simulink library "halout"  (R2021b)
settings: Solver=VariableStepAuto  StartTime=0.0  StopTime=10.0  RelTol=1e-3
undefined symbols (not defined in the file): C_TASK_5MS_S, FALSE, KHAL_CAN1TxReq_flg, KHAL_CAN2TxReq_flg, KHAL_CAN3FD3VCU1toNIDECTxReq_flg, KHAL_CAN3FD3VCU1TxReq_flg, KHAL_CAN3FD3VCU2E2E_flg, KHAL_CAN3FD3VCU2toNIDECE2E_flg, KHAL_CAN3FD3VCU2toNIDECTxReq_flg, KHAL_CAN3FD3VCU2TxReq_flg, KHAL_CAN3TxReq_flg, KHAL_CAN4FD4CE1000E2E_flg, KHAL_CAN4FD4CE1000TxReq_flg, KHAL_CAN4TxReq_flg, KHAL_CAN5TxReq_flg, KHAL_CAN7TxReq_flg, ONE_INT, TRUE, ZERO_INT
libraries: FVT_lib x258, simulink x115
(part 1 of 17)
settings Model: Creator=13168  LastModifiedBy=FVT22063
settings SolverCC: AlgebraicLoopSolver=TrustRegion
settings DataIOCC: SaveFormat=Array  SignalLoggingSaveFormat=ModelDataLogs  ReturnWorkspaceOutputs=off
settings OptimizationCC: BlockReduction=off  BooleanDataType=off
settings DebuggingCC: SaveWithParameterizedLinksMsg=none  UnderspecifiedInitializationDetection=Classic  MergeDetectMultiDrivingBlocksExec=none  SignalResolutionControl=TryResolveAllWithWarning  SFMachineParentedDataDiag=warning
settings HardwareCC: TargetUnknown=on
settings ModelReferenceCC: PropagateSignalLabelsOutOfModel=off
settings ConfigComp: CovMetricSettings=dw  CovSaveCumulativeToWorkspaceVar=on  CovSaveSingleToWorkspaceVar=on

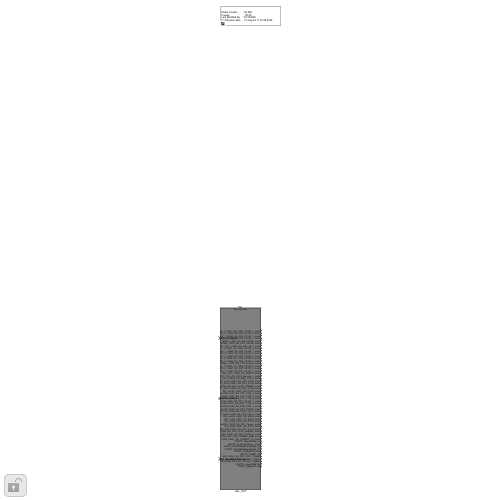
[thumbnail: Simulink's stored preview of the top-level diagram]
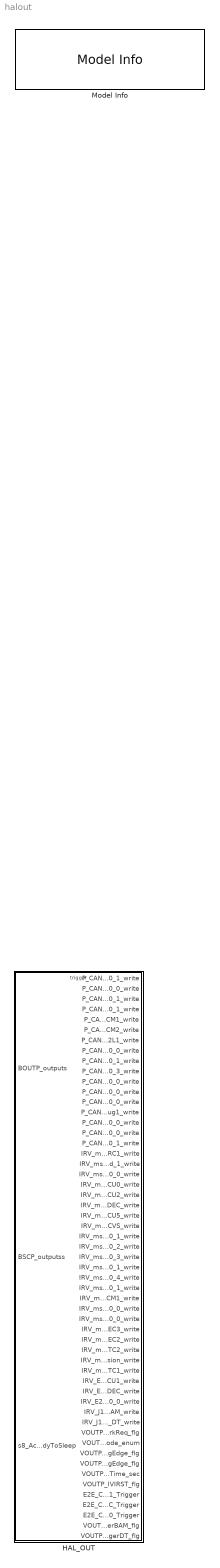
== system halout ==
  HAL_OUT : Subsystem
      settings: RTWSystemCode=Nonreusable function  RTWFcnNameOpts=Use subsystem name  RTWFileNameOpts=Use subsystem name
  Model Info : simulink/Model-Wide Utilities/Model Info  Frame=on  DisplayStringWithTags=|  HorizontalTextAlignment=Left  LeftAlignmentValue=0.02
      | Model Version        : %<ModelVersion>
      | Creator                   : %<Creator>
      | Last Modified By    : %<LastModifiedBy>
      | Modification date    : %<LastModificationDate>

== system halout/HAL_OUT ==
  BOUTP_outputs : Inport  OutDataTypeStr=Bus: BOUTP_outputs
  BSCP_outputss : Inport  Port=2  OutDataTypeStr=Bus:BSCP_outputs
  s8_AcoreReadyToSleep : Inport  Port=3
  trig_hal_out : TriggerPort  TriggerType=function-call  VariantControl=(inherit)
  Bus Selector : BusSelector  OutputSignals=VOUTP_AllCANTxReq_flg
  Bus_Selector : BusSelector  OutputSignals=VOUTP_NetworkReq_flg,VOUTP_SysPowerMode_enum,VOUTP_NvWriteReqRisingEdge_flg,VOUTP_FdcSlpReqRisingEdge_flg,VOUTP_FdcSlpTime_sec,VOUTP_triggerBAM_flg,VOUTP_triggerDT_flg
  CAN1 : Subsystem  TreatAsAtomicUnit=on
  CAN2 : Subsystem  TreatAsAtomicUnit=on
  CAN3 : Subsystem  TreatAsAtomicUnit=on
  CAN4 : Subsystem  TreatAsAtomicUnit=on
  CAN5 : Subsystem  TreatAsAtomicUnit=on
  CAN7 : Subsystem  TreatAsAtomicUnit=on
  CAN_Scheduler : Stateflow chart  TreatAsAtomicUnit=on
  Constant : Constant  Value=KHAL_CAN1TxReq_flg
  Constant1 : Constant  Value=KHAL_CAN2TxReq_flg
  Constant2 : Constant  Value=KHAL_CAN3TxReq_flg
  Constant3 : Constant  Value=KHAL_CAN4TxReq_flg
  Constant4 : Constant  Value=KHAL_CAN5TxReq_flg
  Constant5 : Constant  Value=KHAL_CAN7TxReq_flg
  Ground : Ground
  P_CAN1_GW1_C1000_1_CAN1_SG_GW1_C1000_1_write : Outport  OutDataTypeStr=Bus: DT_CAN1_SG_GW1_C1000_1
  P_CAN2_FD2_CE100_0_CAN2_SG_FD2_CE100_0_write : Outport  Port=2  OutDataTypeStr=Bus: DT_CAN2_SG_FD2_CE100_0
  P_CAN2_FD2_CE100_1_CAN2_SG_FD2_CE100_1_write : Outport  Port=3  OutDataTypeStr=Bus: DT_CAN2_SG_FD2_CE100_1
  P_CAN2_FD2_CE200_1_CAN2_SG_FD2_CE200_1_write : Outport  Port=4  OutDataTypeStr=Bus: DT_CAN2_SG_FD2_CE200_1
  P_CAN3_FD3_BCM1_CAN3_SG_FD3_BCM1_write : Outport  Port=5  OutDataTypeStr=Bus: DT_CAN3_SG_FD3_BCM1
  P_CAN3_FD3_THCM2_CAN3_SG_FD3_THCM2_write : Outport  Port=6  OutDataTypeStr=Bus: DT_CAN3_SG_FD3_THCM2
  P_CAN3_FD3_V2L1_CAN3_SG_FD3_V2L1_write : Outport  Port=7  OutDataTypeStr=Bus: DT_CAN3_SG_FD3_V2L1
  P_CAN3_GW3_CE100_0_CAN3_SG_GW3_CE100_0_write : Outport  Port=8  OutDataTypeStr=Bus: DT_CAN3_SG_GW3_CE100_0
  P_CAN4_FD4_CE100_1_CAN4_SG_FD4_CE100_1_write : Outport  Port=9  OutDataTypeStr=Bus: DT_CAN4_SG_FD4_CE100_1
  P_CAN4_FD4_CE100_3_CAN4_SG_FD4_CE100_3_write : Outport  Port=10  OutDataTypeStr=Bus: DT_CAN4_SG_FD4_CE100_3
  P_CAN4_FD4_CE200_0_CAN4_SG_FD4_CE200_0_write : Outport  Port=11  OutDataTypeStr=Bus: DT_CAN4_SG_FD4_CE200_0
  P_CAN4_GW4_CE100_0_CAN4_SG_GW4_CE100_0_write : Outport  Port=12  OutDataTypeStr=Bus: DT_CAN4_SG_GW4_CE100_0
  P_CAN5_FD5_CE100_0_CAN5_SG_FD5_CE100_0_write : Outport  Port=13  OutDataTypeStr=Bus: DT_CAN5_SG_FD5_CE100_0
  P_CAN5_FD5_Debug1_CAN5_SG_FD5_Debug1_write : Outport  Port=14  OutDataTypeStr=Bus: DT_CAN5_SG_FD5_Debug1
  P_CAN5_GW5_CE100_0_CAN5_SG_GW5_CE100_0_write : Outport  Port=15  OutDataTypeStr=Bus: DT_CAN5_SG_GW5_CE100_0
  P_CAN7_FD7_CE100_0_CAN7_SG_FD7_CE100_0_write : Outport  Port=16  OutDataTypeStr=Bus: DT_CAN7_SG_FD7_CE100_0
  P_CAN7_FD7_CE100_1_CAN7_SG_FD7_CE100_1_write : Outport  Port=17  OutDataTypeStr=Bus: DT_CAN7_SG_FD7_CE100_1
  IRV_ms10_CAN1_SG_EMRC1_write : Outport  Port=18  OutDataTypeStr=Bus: DT_CAN1_SG_EMRC1
  IRV_ms10_CAN1_SG_VCU_PDU_Demand_1_write : Outport  Port=19  OutDataTypeStr=Bus: DT_CAN1_SG_VCU_PDU_Demand_1
  IRV_ms10_CAN2_SG_GW2_C10_0_write : Outport  Port=20  OutDataTypeStr=Bus: DT_CAN2_SG_GW2_C10_0
  IRV_ms10_CAN3_SG_FD3_VCU0_write : Outport  Port=21  OutDataTypeStr=Bus: DT_CAN3_SG_FD3_VCU0
  IRV_ms10_CAN3_SG_FD3_VCU2_write : Outport  Port=22  OutDataTypeStr=Bus: DT_CAN3_SG_FD3_VCU2
  IRV_ms10_CAN3_SG_FD3_VCU2_toNIDEC_write : Outport  Port=23  OutDataTypeStr=Bus: DT_CAN3_SG_FD3_VCU2_toNIDEC
  IRV_ms10_CAN3_SG_FD3_VCU5_write : Outport  Port=24  OutDataTypeStr=Bus: DT_CAN3_SG_FD3_VCU5
  IRV_ms100_CAN1_SG_CCVS_write : Outport  Port=25  OutDataTypeStr=Bus: DT_CAN1_SG_CCVS
  IRV_ms100_CAN1_SG_FD1_C100_1_write : Outport  Port=26  OutDataTypeStr=Bus: DT_CAN1_SG_FD1_C100_1
  IRV_ms100_CAN1_SG_FD1_C100_2_write : Outport  Port=27  OutDataTypeStr=Bus: DT_CAN1_SG_FD1_C100_2
  IRV_ms100_CAN1_SG_FD1_C100_3_write : Outport  Port=28  OutDataTypeStr=Bus: DT_CAN1_SG_FD1_C100_3
  IRV_ms100_CAN1_SG_FD1_CE100_1_write : Outport  Port=29  OutDataTypeStr=Bus: DT_CAN1_SG_FD1_CE100_1
  IRV_ms100_CAN1_SG_GW1_C100_4_write : Outport  Port=30  OutDataTypeStr=Bus: DT_CAN1_SG_GW1_C100_4
  IRV_ms100_CAN2_SG_FD2_C200_1_write : Outport  Port=31  OutDataTypeStr=Bus: DT_CAN2_SG_FD2_C200_1
  IRV_ms100_CAN3_SG_FD3_THCM1_write : Outport  Port=32  OutDataTypeStr=Bus: DT_CAN3_SG_FD3_THCM1
  IRV_ms100_CAN4_SG_FD4_C100_0_write : Outport  Port=33  OutDataTypeStr=Bus: DT_CAN4_SG_FD4_C100_0
  IRV_ms20_CAN2_SG_FD2_C20_0_write : Outport  Port=34  OutDataTypeStr=Bus: DT_CAN2_SG_FD2_C20_0
  IRV_ms250_CAN1_SG_EEC3_write : Outport  Port=35  OutDataTypeStr=Bus: DT_CAN1_SG_EEC3
  IRV_ms50_CAN1_SG_EEC2_write : Outport  Port=36  OutDataTypeStr=Bus: DT_CAN1_SG_EEC2
  IRV_ms50_CAN1_SG_ETC2_write : Outport  Port=37  OutDataTypeStr=Bus: DT_CAN1_SG_ETC2
  IRV_ms5000_CAN2_SG_FD2_Version_write : Outport  Port=38  OutDataTypeStr=Bus: DT_CAN2_SG_FD2_Version
  IRV_ms80_CAN1_SG_ETC1_write : Outport  Port=39  OutDataTypeStr=Bus: DT_CAN1_SG_ETC1
  IRV_E2E_CAN3_SG_FD3_VCU1_write : Outport  Port=40  OutDataTypeStr=Bus: DT_CAN3_SG_FD3_VCU1
  IRV_E2E_CAN3_SG_FD3_VCU1_toNIDEC_write : Outport  Port=41  OutDataTypeStr=Bus: DT_CAN3_SG_FD3_VCU1_toNIDEC
  IRV_E2E_CAN4_SG_FD4_CE100_0_write : Outport  Port=42  OutDataTypeStr=Bus: DT_CAN4_SG_FD4_CE100_0
  IRV_J1939_CAN1_SG_CFGEM1_BAM_write : Outport  Port=43  OutDataTypeStr=Bus: DT_CAN1_SG_CFGEM1_BAM
  IRV_J1939_CAN1_SG_CFGEM1_DT_write : Outport  Port=44  OutDataTypeStr=Bus: DT_CAN1_SG_CFGEM1_DT
  VOUTP_NetworkReq_flg : Outport  Port=45
  VOUTP_SysPowerMode_enum : Outport  Port=46
  VOUTP_NvWriteReqRisingEdge_flg : Outport  Port=47
  VOUTP_FdcSlpReqRisingEdge_flg : Outport  Port=48
  VOUTP_FdcSlpTime_sec : Outport  Port=49
  VOUTP_IVIRST_flg : Outport  Port=50
  E2E_CAN3_SG_FD3_VCU1_Trigger : Outport  Port=51
  E2E_CAN3_SG_FD3_VCU1_toNIDEC_Trigger : Outport  Port=52
  E2E_CAN4_SG_FD4_CE100_0_Trigger : Outport  Port=53
  VOUTP_triggerBAM_flg : Outport  Port=54
  VOUTP_triggerDT_flg : Outport  Port=55
  wires:
  BSCP_outputss/1 -> [BSCP_outputs]
  BOUTP_outputs/1 -> [BOUTP_outputs]
  Bus Selector/1 -> CAN_Scheduler/7(VOUTP_ALLCANTxReq_flg)  "<VOUTP_AllCANTxReq_flg>"
  [BOUTP_outputs] -> Bus Selector/1
  Constant1/1 -> CAN_Scheduler/2(KHAL_CAN2TxReq_flg)
  Constant3/1 -> CAN_Scheduler/4(KHAL_CAN4TxReq_flg)
  CAN_Scheduler/1(trig_can1()) -> [trig_can1]
  CAN_Scheduler/2(trig_can2()) -> [trig_can2]
  Constant/1 -> CAN_Scheduler/1(KHAL_CAN1TxReq_flg)
  CAN_Scheduler/4(trig_can4()) -> [trig_can4]
  CAN_Scheduler/5(trig_can5()) -> [trig_can5]
  Constant4/1 -> CAN_Scheduler/5(KHAL_CAN5TxReq_flg)
  Constant2/1 -> CAN_Scheduler/3(KHAL_CAN3TxReq_flg)
  CAN_Scheduler/3(trig_can3()) -> [trig_can3]
  [trig_can1] -> CAN1/Trigger
  [trig_can4] -> CAN4/Trigger
  [trig_can5] -> CAN5/Trigger
  [trig_can2] -> CAN2/Trigger
  [trig_can3] -> CAN3/Trigger
  Constant5/1 -> CAN_Scheduler/6(KHAL_CAN6TxReq_flg)
  CAN_Scheduler/6(trig_can6()) -> [trig_can6]
  [trig_can6] -> CAN7/Trigger
  [BSCP_outputs] -> CAN7/2(BSCP_outputs)
  [BOUTP_outputs] -> CAN7/1(BOUTP_outputs)
  [BSCP_outputs] -> CAN5/2(BSCP_outputs)
  CAN4/2(E2E_CAN4_SG_FD4_CE100_0_Trigger) -> E2E_CAN4_SG_FD4_CE100_0_Trigger/1
  CAN3/6(E2E_CAN3_SG_FD3_VCU1_Trigger) -> E2E_CAN3_SG_FD3_VCU1_Trigger/1
  CAN3/8(E2E_CAN3_SG_FD3_VCU1_toNIDEC_Trigger) -> E2E_CAN3_SG_FD3_VCU1_toNIDEC_Trigger/1
  [BSCP_outputs] -> CAN4/2(BSCP_outputs)
  [BOUTP_outputs] -> CAN1/1(BOUTP_outputs)
  Bus_Selector/5 -> VOUTP_FdcSlpTime_sec/1  "<VOUTP_FdcSlpTime_sec>"
  [BSCP_outputs] -> CAN2/2(BSCP_outputs)
  Bus_Selector/3 -> VOUTP_NvWriteReqRisingEdge_flg/1  "<VOUTP_NvWriteReqRisingEdge_flg>"
  Bus_Selector/2 -> VOUTP_SysPowerMode_enum/1  "<VOUTP_SysPowerMode_enum>"
  CAN1/3(DT_CAN1_SG_CFGEM1_DT) -> IRV_J1939_CAN1_SG_CFGEM1_DT_write/1
  CAN1/2(DT_CAN1_SG_CFGEM1_BAM) -> IRV_J1939_CAN1_SG_CFGEM1_BAM_write/1
  CAN4/3(DT_CAN4_SG_FD4_CE100_0) -> IRV_E2E_CAN4_SG_FD4_CE100_0_write/1
  [BOUTP_outputs] -> Bus_Selector/1
  [BOUTP_outputs] -> CAN2/1(BOUTP_outputs)
  CAN4/1(DT_CAN4_SG_FD4_C100_0) -> IRV_ms100_CAN4_SG_FD4_C100_0_write/1
  CAN2/1(DT_CAN2_SG_FD2_C200_1) -> IRV_ms100_CAN2_SG_FD2_C200_1_write/1
  CAN1/8(DT_CAN1_SG_ETC2) -> IRV_ms50_CAN1_SG_ETC2_write/1
  CAN1/14(DT_CAN1_SG_GW1_C100_4) -> IRV_ms100_CAN1_SG_GW1_C100_4_write/1
  CAN1/11(DT_CAN1_SG_FD1_C100_3) -> IRV_ms100_CAN1_SG_FD1_C100_3_write/1
  [BOUTP_outputs] -> CAN5/1(BOUTP_outputs)
  CAN1/10(DT_CAN1_SG_FD1_C100_2) -> IRV_ms100_CAN1_SG_FD1_C100_2_write/1
  [BSCP_outputs] -> CAN3/2(BSCP_outputs)
  [BOUTP_outputs] -> CAN4/1(BOUTP_outputs)
  [BOUTP_outputs] -> CAN3/1(BOUTP_outputs)
  CAN1/12(DT_CAN1_SG_FD1_CE100_1) -> IRV_ms100_CAN1_SG_FD1_CE100_1_write/1
  CAN1/1(DT_CAN1_SG_CCVS) -> IRV_ms100_CAN1_SG_CCVS_write/1
  CAN3/12(DT_CAN3_SG_FD3_VCU5) -> IRV_ms10_CAN3_SG_FD3_VCU5_write/1
  CAN3/11(DT_CAN3_SG_FD3_VCU2_toNIDEC) -> IRV_ms10_CAN3_SG_FD3_VCU2_toNIDEC_write/1
  CAN2/6(DT_CAN2_SG_FD2_Version) -> IRV_ms5000_CAN2_SG_FD2_Version_write/1
  CAN3/10(DT_CAN3_SG_FD3_VCU2) -> IRV_ms10_CAN3_SG_FD3_VCU2_write/1
  CAN1/7(DT_CAN1_SG_ETC1) -> IRV_ms80_CAN1_SG_ETC1_write/1
  CAN3/5(DT_CAN3_SG_FD3_VCU0) -> IRV_ms10_CAN3_SG_FD3_VCU0_write/1
  Bus_Selector/4 -> VOUTP_FdcSlpReqRisingEdge_flg/1  "<VOUTP_FdcSlpReqRisingEdge_flg>"
  [BSCP_outputs] -> CAN1/2(BSCP_outputs)
  CAN2/7(DT_CAN2_SG_GW2_C10_0) -> IRV_ms10_CAN2_SG_GW2_C10_0_write/1
  CAN1/6(DT_CAN1_SG_EMRC1) -> IRV_ms10_CAN1_SG_EMRC1_write/1
  CAN7/2(DT_CAN7_SG_FD7_CE100_1) -> P_CAN7_FD7_CE100_1_CAN7_SG_FD7_CE100_1_write/1
  CAN5/3(DT_CAN5_SG_GW5_CE100_0) -> P_CAN5_GW5_CE100_0_CAN5_SG_GW5_CE100_0_write/1
  CAN7/1(DT_CAN7_SG_FD7_CE100_0) -> P_CAN7_FD7_CE100_0_CAN7_SG_FD7_CE100_0_write/1
  CAN5/2(DT_CAN5_SG_FD5_Debug1) -> P_CAN5_FD5_Debug1_CAN5_SG_FD5_Debug1_write/1
  CAN3/9(DT_CAN3_SG_FD3_VCU1_toNIDEC) -> IRV_E2E_CAN3_SG_FD3_VCU1_toNIDEC_write/1
  CAN5/1(DT_CAN5_SG_FD5_CE100_0) -> P_CAN5_FD5_CE100_0_CAN5_SG_FD5_CE100_0_write/1
  CAN4/7(DT_CAN4_SG_GW4_CE100_0) -> P_CAN4_GW4_CE100_0_CAN4_SG_GW4_CE100_0_write/1
  CAN3/7(DT_CAN3_SG_FD3_VCU1) -> IRV_E2E_CAN3_SG_FD3_VCU1_write/1
  CAN4/6(DT_CAN4_SG_FD4_CE200_0) -> P_CAN4_FD4_CE200_0_CAN4_SG_FD4_CE200_0_write/1
  CAN2/2(DT_CAN2_SG_FD2_C20_0) -> IRV_ms20_CAN2_SG_FD2_C20_0_write/1
  CAN1/4(DT_CAN1_SG_EEC2) -> IRV_ms50_CAN1_SG_EEC2_write/1
  CAN4/5(DT_CAN4_SG_FD4_CE100_3) -> P_CAN4_FD4_CE100_3_CAN4_SG_FD4_CE100_3_write/1
  CAN1/9(DT_CAN1_SG_FD1_C100_1) -> IRV_ms100_CAN1_SG_FD1_C100_1_write/1
  CAN4/4(DT_CAN4_SG_FD4_CE100_1) -> P_CAN4_FD4_CE100_1_CAN4_SG_FD4_CE100_1_write/1
  CAN3/13(DT_CAN3_SG_GW3_CE100_0) -> P_CAN3_GW3_CE100_0_CAN3_SG_GW3_CE100_0_write/1
  CAN3/3(DT_CAN3_SG_FD3_THCM2) -> P_CAN3_FD3_THCM2_CAN3_SG_FD3_THCM2_write/1
  CAN3/4(DT_CAN3_SG_FD3_V2L1) -> P_CAN3_FD3_V2L1_CAN3_SG_FD3_V2L1_write/1
  CAN1/5(DT_CAN1_SG_EEC3) -> IRV_ms250_CAN1_SG_EEC3_write/1
  CAN3/1(DT_CAN3_SG_FD3_BCM1) -> P_CAN3_FD3_BCM1_CAN3_SG_FD3_BCM1_write/1
  CAN2/3(DT_CAN2_SG_FD2_CE100_0) -> P_CAN2_FD2_CE100_0_CAN2_SG_FD2_CE100_0_write/1
  Bus_Selector/1 -> VOUTP_NetworkReq_flg/1  "<VOUTP_NetworkReq_flg>"
  CAN3/2(DT_CAN3_SG_FD3_THCM1) -> IRV_ms100_CAN3_SG_FD3_THCM1_write/1
  CAN2/4(DT_CAN2_SG_FD2_CE100_1) -> P_CAN2_FD2_CE100_1_CAN2_SG_FD2_CE100_1_write/1
  CAN2/5(DT_CAN2_SG_FD2_CE200_1) -> P_CAN2_FD2_CE200_1_CAN2_SG_FD2_CE200_1_write/1
  CAN1/15(DT_CAN1_SG_VCU_PDU_Demand_1) -> IRV_ms10_CAN1_SG_VCU_PDU_Demand_1_write/1
  CAN1/13(DT_CAN1_SG_GW1_C1000_1) -> P_CAN1_GW1_C1000_1_CAN1_SG_GW1_C1000_1_write/1
  s8_AcoreReadyToSleep/1 -> CAN3/3(s8_AcoreReadyToSleep)
  Bus_Selector/6 -> VOUTP_triggerBAM_flg/1  "<VOUTP_triggerBAM_flg>"
  Bus_Selector/7 -> VOUTP_triggerDT_flg/1  "<VOUTP_triggerDT_flg>"
  Ground/1 -> VOUTP_IVIRST_flg/1

== system halout/HAL_OUT/CAN1 ==
  BOUTP_outputs : Inport  OutDataTypeStr=Bus: BOUTP_outputs
  BSCP_outputs : Inport  Port=2  OutDataTypeStr=Bus: BSCP_outputs
  Trigger : TriggerPort  TriggerType=function-call  VariantControl=(inherit)
  CCVS_0x18FEF100 : Subsystem
  CFGEM1_BAM_0x18ECFFEF : Subsystem
  CFGEM1_DT_0x18EBFFEF : Subsystem
  EEC2_0xCF00300 : Subsystem
  EEC3_0x18FEDFEF : Subsystem
  EMRC1_0x18FF20EF : Subsystem
  ETC1_0x18F00203 : Subsystem
  ETC2_0x18F00503 : Subsystem
  FD1_C100_1_0x18FF602B : Subsystem
  FD1_C100_2_0x18FE4A03 : Subsystem
  FD1_C100_3_0xCF103D0 : Subsystem
  FD1_CE100_1_0x18FE4EEC : Subsystem
  GW1_C1000_1_0x18E0FF21 : Subsystem
  GW1_C100_4_0x18FDA521 : Subsystem
  VCU_PDU_Demand_1_0xCF101D0 : Subsystem
  DT_CAN1_SG_CCVS : Outport  OutDataTypeStr=Bus: DT_CAN1_SG_CCVS
  DT_CAN1_SG_CFGEM1_BAM : Outport  Port=2  OutDataTypeStr=Bus: DT_CAN1_SG_CFGEM1_BAM
  DT_CAN1_SG_CFGEM1_DT : Outport  Port=3  OutDataTypeStr=Bus: DT_CAN1_SG_CFGEM1_DT
  DT_CAN1_SG_EEC2 : Outport  Port=4  OutDataTypeStr=Bus: DT_CAN1_SG_EEC2
  DT_CAN1_SG_EEC3 : Outport  Port=5  OutDataTypeStr=Bus: DT_CAN1_SG_EEC3
  DT_CAN1_SG_EMRC1 : Outport  Port=6  OutDataTypeStr=Bus: DT_CAN1_SG_EMRC1
  DT_CAN1_SG_ETC1 : Outport  Port=7  OutDataTypeStr=Bus: DT_CAN1_SG_ETC1
  DT_CAN1_SG_ETC2 : Outport  Port=8  OutDataTypeStr=Bus: DT_CAN1_SG_ETC2
  DT_CAN1_SG_FD1_C100_1 : Outport  Port=9  OutDataTypeStr=Bus: DT_CAN1_SG_FD1_C100_1
  DT_CAN1_SG_FD1_C100_2 : Outport  Port=10  OutDataTypeStr=Bus: DT_CAN1_SG_FD1_C100_2
  DT_CAN1_SG_FD1_C100_3 : Outport  Port=11  OutDataTypeStr=Bus: DT_CAN1_SG_FD1_C100_3
  DT_CAN1_SG_FD1_CE100_1 : Outport  Port=12  OutDataTypeStr=Bus: DT_CAN1_SG_FD1_CE100_1
  DT_CAN1_SG_GW1_C1000_1 : Outport  Port=13  OutDataTypeStr=Bus: DT_CAN1_SG_GW1_C1000_1
  DT_CAN1_SG_GW1_C100_4 : Outport  Port=14  OutDataTypeStr=Bus: DT_CAN1_SG_GW1_C100_4
  DT_CAN1_SG_VCU_PDU_Demand_1 : Outport  Port=15  OutDataTypeStr=Bus: DT_CAN1_SG_VCU_PDU_Demand_1
  wires:
  BOUTP_outputs/1 -> [BOUTP_outputs]
  BSCP_outputs/1 -> [BSCP_outputs]
  [BSCP_outputs] -> CCVS_0x18FEF100/1(BSCP_outputs)
  [BOUTP_outputs] -> CCVS_0x18FEF100/2(BOUTP_outputs)
  CCVS_0x18FEF100/1(CCVS) -> DT_CAN1_SG_CCVS/1
  [BSCP_outputs] -> CFGEM1_BAM_0x18ECFFEF/1(BSCP_outputs)
  [BOUTP_outputs] -> CFGEM1_BAM_0x18ECFFEF/2(BOUTP_outputs)
  CFGEM1_BAM_0x18ECFFEF/1(CFGEM1_BAM) -> DT_CAN1_SG_CFGEM1_BAM/1
  [BSCP_outputs] -> CFGEM1_DT_0x18EBFFEF/1(BSCP_outputs)
  [BOUTP_outputs] -> CFGEM1_DT_0x18EBFFEF/2(BOUTP_outputs)
  CFGEM1_DT_0x18EBFFEF/1(CFGEM1_DT) -> DT_CAN1_SG_CFGEM1_DT/1
  [BSCP_outputs] -> EEC2_0xCF00300/1(BSCP_outputs)
  [BOUTP_outputs] -> EEC2_0xCF00300/2(BOUTP_outputs)
  EEC2_0xCF00300/1(EEC2) -> DT_CAN1_SG_EEC2/1
  [BSCP_outputs] -> EEC3_0x18FEDFEF/1(BSCP_outputs)
  [BOUTP_outputs] -> EEC3_0x18FEDFEF/2(BOUTP_outputs)
  EEC3_0x18FEDFEF/1(EEC3) -> DT_CAN1_SG_EEC3/1
  [BSCP_outputs] -> EMRC1_0x18FF20EF/1(BSCP_outputs)
  [BOUTP_outputs] -> EMRC1_0x18FF20EF/2(BOUTP_outputs)
  EMRC1_0x18FF20EF/1(EMRC1) -> DT_CAN1_SG_EMRC1/1
  [BSCP_outputs] -> ETC1_0x18F00203/1(BSCP_outputs)
  [BOUTP_outputs] -> ETC1_0x18F00203/2(BOUTP_outputs)
  ETC1_0x18F00203/1(ETC1) -> DT_CAN1_SG_ETC1/1
  [BSCP_outputs] -> ETC2_0x18F00503/1(BSCP_outputs)
  [BOUTP_outputs] -> ETC2_0x18F00503/2(BOUTP_outputs)
  ETC2_0x18F00503/1(ETC2) -> DT_CAN1_SG_ETC2/1
  [BSCP_outputs] -> FD1_C100_1_0x18FF602B/1(BSCP_outputs)
  [BOUTP_outputs] -> FD1_C100_1_0x18FF602B/2(BOUTP_outputs)
  FD1_C100_1_0x18FF602B/1(FD1_C100_1) -> DT_CAN1_SG_FD1_C100_1/1
  [BSCP_outputs] -> FD1_C100_2_0x18FE4A03/1(BSCP_outputs)
  [BOUTP_outputs] -> FD1_C100_2_0x18FE4A03/2(BOUTP_outputs)
  FD1_C100_2_0x18FE4A03/1(FD1_C100_2) -> DT_CAN1_SG_FD1_C100_2/1
  [BSCP_outputs] -> FD1_C100_3_0xCF103D0/1(BSCP_outputs)
  [BOUTP_outputs] -> FD1_C100_3_0xCF103D0/2(BOUTP_outputs)
  FD1_C100_3_0xCF103D0/1(FD1_C100_3) -> DT_CAN1_SG_FD1_C100_3/1
  [BSCP_outputs] -> FD1_CE100_1_0x18FE4EEC/1(BSCP_outputs)
  [BOUTP_outputs] -> FD1_CE100_1_0x18FE4EEC/2(BOUTP_outputs)
  FD1_CE100_1_0x18FE4EEC/1(FD1_CE100_1) -> DT_CAN1_SG_FD1_CE100_1/1
  [BSCP_outputs] -> GW1_C1000_1_0x18E0FF21/1(BSCP_outputs)
  [BOUTP_outputs] -> GW1_C1000_1_0x18E0FF21/2(BOUTP_outputs)
  GW1_C1000_1_0x18E0FF21/1(GW1_C1000_1) -> DT_CAN1_SG_GW1_C1000_1/1
  [BSCP_outputs] -> GW1_C100_4_0x18FDA521/1(BSCP_outputs)
  [BOUTP_outputs] -> GW1_C100_4_0x18FDA521/2(BOUTP_outputs)
  GW1_C100_4_0x18FDA521/1(GW1_C100_4) -> DT_CAN1_SG_GW1_C100_4/1
  [BSCP_outputs] -> VCU_PDU_Demand_1_0xCF101D0/1(BSCP_outputs)
  [BOUTP_outputs] -> VCU_PDU_Demand_1_0xCF101D0/2(BOUTP_outputs)
  VCU_PDU_Demand_1_0xCF101D0/1(VCU_PDU_Demand_1) -> DT_CAN1_SG_VCU_PDU_Demand_1/1

== system halout/HAL_OUT/CAN2 ==
  BOUTP_outputs : Inport  OutDataTypeStr=Bus: BOUTP_outputs
  BSCP_outputs : Inport  Port=2  OutDataTypeStr=Bus: BSCP_outputs
  Trigger : TriggerPort  TriggerType=function-call  VariantControl=(inherit)
  FD2_C200_1_0x18F001EF : Subsystem
  FD2_C20_0_0x210 : Subsystem
  FD2_CE100_0_0x117 : Subsystem
  FD2_CE100_1_0x202 : Subsystem
  FD2_CE200_1_0x435 : Subsystem
  FD2_Version_0x3C3 : Subsystem
  GW2_C10_0_0x1B3 : Subsystem
  DT_CAN2_SG_FD2_C200_1 : Outport  OutDataTypeStr=Bus: DT_CAN2_SG_FD2_C200_1
  DT_CAN2_SG_FD2_C20_0 : Outport  Port=2  OutDataTypeStr=Bus: DT_CAN2_SG_FD2_C20_0
  DT_CAN2_SG_FD2_CE100_0 : Outport  Port=3  OutDataTypeStr=Bus: DT_CAN2_SG_FD2_CE100_0
  DT_CAN2_SG_FD2_CE100_1 : Outport  Port=4  OutDataTypeStr=Bus: DT_CAN2_SG_FD2_CE100_1
  DT_CAN2_SG_FD2_CE200_1 : Outport  Port=5  OutDataTypeStr=Bus: DT_CAN2_SG_FD2_CE200_1
  DT_CAN2_SG_FD2_Version : Outport  Port=6  OutDataTypeStr=Bus: DT_CAN2_SG_FD2_Version
  DT_CAN2_SG_GW2_C10_0 : Outport  Port=7  OutDataTypeStr=Bus: DT_CAN2_SG_GW2_C10_0
  wires:
  BOUTP_outputs/1 -> [BOUTP_outputs]
  BSCP_outputs/1 -> [BSCP_outputs]
  [BSCP_outputs] -> FD2_C200_1_0x18F001EF/1(BSCP_outputs)
  [BOUTP_outputs] -> FD2_C200_1_0x18F001EF/2(BOUTP_outputs)
  FD2_C200_1_0x18F001EF/1(FD2_C200_1) -> DT_CAN2_SG_FD2_C200_1/1
  [BSCP_outputs] -> FD2_C20_0_0x210/1(BSCP_outputs)
  [BOUTP_outputs] -> FD2_C20_0_0x210/2(BOUTP_outputs)
  FD2_C20_0_0x210/1(FD2_C20_0) -> DT_CAN2_SG_FD2_C20_0/1
  [BSCP_outputs] -> FD2_CE100_0_0x117/1(BSCP_outputs)
  [BOUTP_outputs] -> FD2_CE100_0_0x117/2(BOUTP_outputs)
  FD2_CE100_0_0x117/1(FD2_CE100_0) -> DT_CAN2_SG_FD2_CE100_0/1
  [BSCP_outputs] -> FD2_CE100_1_0x202/1(BSCP_outputs)
  [BOUTP_outputs] -> FD2_CE100_1_0x202/2(BOUTP_outputs)
  FD2_CE100_1_0x202/1(FD2_CE100_1) -> DT_CAN2_SG_FD2_CE100_1/1
  [BSCP_outputs] -> FD2_CE200_1_0x435/1(BSCP_outputs)
  [BOUTP_outputs] -> FD2_CE200_1_0x435/2(BOUTP_outputs)
  FD2_CE200_1_0x435/1(FD2_CE200_1) -> DT_CAN2_SG_FD2_CE200_1/1
  [BSCP_outputs] -> FD2_Version_0x3C3/1(BSCP_outputs)
  [BOUTP_outputs] -> FD2_Version_0x3C3/2(BOUTP_outputs)
  FD2_Version_0x3C3/1(FD2_Version) -> DT_CAN2_SG_FD2_Version/1
  [BSCP_outputs] -> GW2_C10_0_0x1B3/1(BSCP_outputs)
  [BOUTP_outputs] -> GW2_C10_0_0x1B3/2(BOUTP_outputs)
  GW2_C10_0_0x1B3/1(GW2_C10_0) -> DT_CAN2_SG_GW2_C10_0/1

== system halout/HAL_OUT/CAN3 ==
  BOUTP_outputs : Inport  OutDataTypeStr=Bus: BOUTP_outputs
  BSCP_outputs : Inport  Port=2  OutDataTypeStr=Bus: BSCP_outputs
  s8_AcoreReadyToSleep : Inport  Port=3
  Trigger : TriggerPort  TriggerType=function-call  VariantControl=(inherit)
  Constant : Constant  Value=KHAL_CAN3FD3VCU1TxReq_flg
  Constant1 : Constant  Value=KHAL_CAN3FD3VCU1toNIDECTxReq_flg
  Constant2 : Constant  Value=KHAL_CAN3FD3VCU2TxReq_flg
  Constant3 : Constant  Value=KHAL_CAN3FD3VCU2toNIDECTxReq_flg
  FD3_BCM1_0x216 : Subsystem
  FD3_THCM1_0x182 : Subsystem
  FD3_THCM2_0x186 : Subsystem
  FD3_V2L1_0x374 : Subsystem
  FD3_VCU0_0x1F0 : Subsystem
  FD3_VCU1_0x115 : Subsystem
  FD3_VCU1_Tx : Subsystem  AncestorBlock=FVT_lib/hal/MsgTxController_CE  mask{CycleTime=100}
      mask prompts: CycleTime "MsgCycleTime_ms"
      mask help: MeasumentTrigerTime
      mask Display: fprintf('Tx Method: CE\nMsg Cycletime ms: %3.0f', CycleTime);
  FD3_VCU1_toNIDEC_0x116 : Subsystem
  FD3_VCU1_toNIDEC_Tx : Subsystem  AncestorBlock=FVT_lib/hal/MsgTxController_CE  mask{CycleTime=100}
      mask prompts: CycleTime "MsgCycleTime_ms"
      mask help: MeasumentTrigerTime
      mask Display: fprintf('Tx Method: CE\nMsg Cycletime ms: %3.0f', CycleTime);
  FD3_VCU2_0x153 : Subsystem  TreatAsAtomicUnit=on
  FD3_VCU2_Tx : Subsystem  AncestorBlock=FVT_lib/hal/MsgTxController  mask{CycleTime=10}
      mask prompts: CycleTime "MsgCycleTime_ms"
      mask help: MeasumentTrigerTime
      mask Display: fprintf('Tx Method: Cycle\nMsg Cycletime ms: %3.0f', CycleTime);
  FD3_VCU2_toNIDEC_0x154 : Subsystem  TreatAsAtomicUnit=on
  FD3_VCU2_toNIDEC_Tx : Subsystem  AncestorBlock=FVT_lib/hal/MsgTxController  mask{CycleTime=10}
      mask prompts: CycleTime "MsgCycleTime_ms"
      mask help: MeasumentTrigerTime
      mask Display: fprintf('Tx Method: Cycle\nMsg Cycletime ms: %3.0f', CycleTime);
  FD3_VCU5_0x155 : Subsystem
  GW3_CE100_0_0x1C3 : Subsystem
  DT_CAN3_SG_FD3_BCM1 : Outport  OutDataTypeStr=Bus: DT_CAN3_SG_FD3_BCM1
  DT_CAN3_SG_FD3_THCM1 : Outport  Port=2  OutDataTypeStr=Bus: DT_CAN3_SG_FD3_THCM1
  DT_CAN3_SG_FD3_THCM2 : Outport  Port=3  OutDataTypeStr=Bus: DT_CAN3_SG_FD3_THCM2
  DT_CAN3_SG_FD3_V2L1 : Outport  Port=4  OutDataTypeStr=Bus: DT_CAN3_SG_FD3_V2L1
  DT_CAN3_SG_FD3_VCU0 : Outport  Port=5  OutDataTypeStr=Bus: DT_CAN3_SG_FD3_VCU0
  E2E_CAN3_SG_FD3_VCU1_Trigger : Outport  Port=6
  DT_CAN3_SG_FD3_VCU1 : Outport  Port=7  OutDataTypeStr=Bus: DT_CAN3_SG_FD3_VCU1
  E2E_CAN3_SG_FD3_VCU1_toNIDEC_Trigger : Outport  Port=8
  DT_CAN3_SG_FD3_VCU1_toNIDEC : Outport  Port=9  OutDataTypeStr=Bus: DT_CAN3_SG_FD3_VCU1_toNIDEC
  DT_CAN3_SG_FD3_VCU2 : Outport  Port=10  OutDataTypeStr=Bus: DT_CAN3_SG_FD3_VCU2
  DT_CAN3_SG_FD3_VCU2_toNIDEC : Outport  Port=11  OutDataTypeStr=Bus: DT_CAN3_SG_FD3_VCU2_toNIDEC
  DT_CAN3_SG_FD3_VCU5 : Outport  Port=12  OutDataTypeStr=Bus: DT_CAN3_SG_FD3_VCU5
  DT_CAN3_SG_GW3_CE100_0 : Outport  Port=13  OutDataTypeStr=Bus: DT_CAN3_SG_GW3_CE100_0
  wires:
  BOUTP_outputs/1 -> [BOUTP_outputs]
  BSCP_outputs/1 -> [BSCP_outputs]
  [BSCP_outputs] -> FD3_BCM1_0x216/1(BSCP_outputs)
  [BOUTP_outputs] -> FD3_BCM1_0x216/2(BOUTP_outputs)
  FD3_BCM1_0x216/1(FD3_BCM1) -> DT_CAN3_SG_FD3_BCM1/1
  [BSCP_outputs] -> FD3_THCM1_0x182/1(BSCP_outputs)
  [BOUTP_outputs] -> FD3_THCM1_0x182/2(BOUTP_outputs)
  FD3_THCM1_0x182/1(FD3_THCM1) -> DT_CAN3_SG_FD3_THCM1/1
  [BSCP_outputs] -> FD3_THCM2_0x186/1(BSCP_outputs)
  [BOUTP_outputs] -> FD3_THCM2_0x186/2(BOUTP_outputs)
  FD3_THCM2_0x186/1(FD3_THCM2) -> DT_CAN3_SG_FD3_THCM2/1
  [BSCP_outputs] -> FD3_V2L1_0x374/1(BSCP_outputs)
  [BOUTP_outputs] -> FD3_V2L1_0x374/2(BOUTP_outputs)
  FD3_V2L1_0x374/1(FD3_V2L1) -> DT_CAN3_SG_FD3_V2L1/1
  [BSCP_outputs] -> FD3_VCU0_0x1F0/1(BSCP_outputs)
  [BOUTP_outputs] -> FD3_VCU0_0x1F0/2(BOUTP_outputs)
  FD3_VCU0_0x1F0/1(FD3_VCU0) -> DT_CAN3_SG_FD3_VCU0/1
  [BSCP_outputs] -> FD3_VCU1_0x115/1(BSCP_outputs)
  [BOUTP_outputs] -> FD3_VCU1_0x115/2(BOUTP_outputs)
  FD3_VCU1_Tx/1(TxTrigger) -> E2E_CAN3_SG_FD3_VCU1_Trigger/1
  Constant/1 -> FD3_VCU1_Tx/1(TxReq)
  [BSCP_outputs] -> FD3_VCU1_Tx/2(BSCP_outputs)
  [BOUTP_outputs] -> FD3_VCU1_Tx/3(BOUTP_outputs)
  FD3_VCU1_0x115/1(FD3_VCU1) -> DT_CAN3_SG_FD3_VCU1/1
  [BSCP_outputs] -> FD3_VCU1_toNIDEC_0x116/1(BSCP_outputs)
  [BOUTP_outputs] -> FD3_VCU1_toNIDEC_0x116/2(BOUTP_outputs)
  FD3_VCU1_toNIDEC_Tx/1(TxTrigger) -> E2E_CAN3_SG_FD3_VCU1_toNIDEC_Trigger/1
  Constant1/1 -> FD3_VCU1_toNIDEC_Tx/1(TxReq)
  [BSCP_outputs] -> FD3_VCU1_toNIDEC_Tx/2(BSCP_outputs)
  [BOUTP_outputs] -> FD3_VCU1_toNIDEC_Tx/3(BOUTP_outputs)
  FD3_VCU1_toNIDEC_0x116/1(FD3_VCU1_toNIDEC) -> DT_CAN3_SG_FD3_VCU1_toNIDEC/1
  [BSCP_outputs] -> FD3_VCU2_0x153/1(BSCP_outputs)
  [BOUTP_outputs] -> FD3_VCU2_0x153/2(BOUTP_outputs)
  FD3_VCU2_Tx/1(TxTrigger) -> FD3_VCU2_0x153/Trigger
  Constant2/1 -> FD3_VCU2_Tx/1(TxReq)
  FD3_VCU2_0x153/1(FD3_VCU2) -> DT_CAN3_SG_FD3_VCU2/1
  [BSCP_outputs] -> FD3_VCU2_toNIDEC_0x154/1(BSCP_outputs)
  [BOUTP_outputs] -> FD3_VCU2_toNIDEC_0x154/2(BOUTP_outputs)
  FD3_VCU2_toNIDEC_Tx/1(TxTrigger) -> FD3_VCU2_toNIDEC_0x154/Trigger
  Constant3/1 -> FD3_VCU2_toNIDEC_Tx/1(TxReq)
  FD3_VCU2_toNIDEC_0x154/1(FD3_VCU2_toNIDEC) -> DT_CAN3_SG_FD3_VCU2_toNIDEC/1
  [BSCP_outputs] -> FD3_VCU5_0x155/1(BSCP_outputs)
  [BOUTP_outputs] -> FD3_VCU5_0x155/2(BOUTP_outputs)
  FD3_VCU5_0x155/1(FD3_VCU5) -> DT_CAN3_SG_FD3_VCU5/1
  [BSCP_outputs] -> GW3_CE100_0_0x1C3/1(BSCP_outputs)
  [BOUTP_outputs] -> GW3_CE100_0_0x1C3/2(BOUTP_outputs)
  GW3_CE100_0_0x1C3/1(GW3_CE100_0) -> DT_CAN3_SG_GW3_CE100_0/1
  s8_AcoreReadyToSleep/1 -> FD3_VCU0_0x1F0/3(s8_AcoreReadyToSleep)

== system halout/HAL_OUT/CAN4 ==
  BOUTP_outputs : Inport  OutDataTypeStr=Bus: BOUTP_outputs
  BSCP_outputs : Inport  Port=2  OutDataTypeStr=Bus: BSCP_outputs
  Trigger : TriggerPort  TriggerType=function-call  VariantControl=(inherit)
  Constant : Constant  Value=KHAL_CAN4FD4CE1000TxReq_flg
  Detect Change : simulink/Logic and Bit Operations/Detect Change  vinit=0  OutDataTypeStr=boolean
  FD4_C100_0_0x202 : Subsystem
  FD4_CE100_0_0x116 : Subsystem  TreatAsAtomicUnit=on
  FD4_CE100_0_Tx : Subsystem  AncestorBlock=FVT_lib/hal/MsgTxController_CE  mask{CycleTime=100}
      mask prompts: CycleTime "MsgCycleTime_ms"
      mask help: MeasumentTrigerTime
      mask Display: fprintf('Tx Method: CE\nMsg Cycletime ms: %3.0f', CycleTime);
  FD4_CE100_1_0x182 : Subsystem
  FD4_CE100_3_0x201 : Subsystem
  FD4_CE200_0_0x217 : Subsystem
  Function-Call Subsystem : Subsystem  TreatAsAtomicUnit=on
  GW4_CE100_0_0x253 : Subsystem
  Unit Delay : UnitDelay  SampleTime=-1  HasFrameUpgradeWarning=on
  DT_CAN4_SG_FD4_C100_0 : Outport  OutDataTypeStr=Bus: DT_CAN4_SG_FD4_C100_0
  E2E_CAN4_SG_FD4_CE100_0_Trigger : Outport  Port=2
  DT_CAN4_SG_FD4_CE100_0 : Outport  Port=3  OutDataTypeStr=Bus: DT_CAN4_SG_FD4_CE100_0
  DT_CAN4_SG_FD4_CE100_1 : Outport  Port=4  OutDataTypeStr=Bus: DT_CAN4_SG_FD4_CE100_1
  DT_CAN4_SG_FD4_CE100_3 : Outport  Port=5  OutDataTypeStr=Bus: DT_CAN4_SG_FD4_CE100_3
  DT_CAN4_SG_FD4_CE200_0 : Outport  Port=6  OutDataTypeStr=Bus: DT_CAN4_SG_FD4_CE200_0
  DT_CAN4_SG_GW4_CE100_0 : Outport  Port=7  OutDataTypeStr=Bus: DT_CAN4_SG_GW4_CE100_0
  wires:
  BOUTP_outputs/1 -> [BOUTP_outputs]
  BSCP_outputs/1 -> [BSCP_outputs]
  [BSCP_outputs] -> FD4_C100_0_0x202/1(BSCP_outputs)
  [BOUTP_outputs] -> FD4_C100_0_0x202/2(BOUTP_outputs)
  FD4_C100_0_0x202/1(FD4_C100_0) -> DT_CAN4_SG_FD4_C100_0/1
  [BSCP_outputs] -> FD4_CE100_0_0x116/1(BSCP_outputs)
  [BOUTP_outputs] -> FD4_CE100_0_0x116/2(BOUTP_outputs)
  Constant/1 -> FD4_CE100_0_Tx/1(TxReq)
  [BSCP_outputs] -> FD4_CE100_0_Tx/2(BSCP_outputs)
  [BOUTP_outputs] -> FD4_CE100_0_Tx/3(BOUTP_outputs)
  FD4_CE100_0_0x116/1(FD4_CE100_0) -> DT_CAN4_SG_FD4_CE100_0/1
  [BSCP_outputs] -> FD4_CE100_1_0x182/1(BSCP_outputs)
  [BOUTP_outputs] -> FD4_CE100_1_0x182/2(BOUTP_outputs)
  FD4_CE100_1_0x182/1(FD4_CE100_1) -> DT_CAN4_SG_FD4_CE100_1/1
  [BSCP_outputs] -> FD4_CE100_3_0x201/1(BSCP_outputs)
  [BOUTP_outputs] -> FD4_CE100_3_0x201/2(BOUTP_outputs)
  FD4_CE100_3_0x201/1(FD4_CE100_3) -> DT_CAN4_SG_FD4_CE100_3/1
  [BSCP_outputs] -> FD4_CE200_0_0x217/1(BSCP_outputs)
  [BOUTP_outputs] -> FD4_CE200_0_0x217/2(BOUTP_outputs)
  FD4_CE200_0_0x217/1(FD4_CE200_0) -> DT_CAN4_SG_FD4_CE200_0/1
  [BSCP_outputs] -> GW4_CE100_0_0x253/1(BSCP_outputs)
  [BOUTP_outputs] -> GW4_CE100_0_0x253/2(BOUTP_outputs)
  GW4_CE100_0_0x253/1(GW4_CE100_0) -> DT_CAN4_SG_GW4_CE100_0/1
  Function-Call Subsystem/1(TriggerCAN4VCU1_CNT) -> Detect Change/1
  Detect Change/1 -> Unit Delay/1
  Unit Delay/1 -> E2E_CAN4_SG_FD4_CE100_0_Trigger/1
  FD4_CE100_0_Tx/2(TriggerCallCDD) -> Function-Call Subsystem/Trigger
  FD4_CE100_0_Tx/1(TriggerDataUpdate) -> FD4_CE100_0_0x116/Trigger

== system halout/HAL_OUT/CAN5 ==
  BOUTP_outputs : Inport  OutDataTypeStr=Bus: BOUTP_outputs
  BSCP_outputs : Inport  Port=2  OutDataTypeStr=Bus: BSCP_outputs
  Trigger : TriggerPort  TriggerType=function-call  VariantControl=(inherit)
  FD5_CE100_0_0x118 : Subsystem
  FD5_Debug1_0x4D0 : Subsystem
  GW5_CE100_0_0x1C5 : Subsystem
  DT_CAN5_SG_FD5_CE100_0 : Outport  OutDataTypeStr=Bus: DT_CAN5_SG_FD5_CE100_0
  DT_CAN5_SG_FD5_Debug1 : Outport  Port=2  OutDataTypeStr=Bus: DT_CAN5_SG_FD5_Debug1
  DT_CAN5_SG_GW5_CE100_0 : Outport  Port=3  OutDataTypeStr=Bus: DT_CAN5_SG_GW5_CE100_0
  wires:
  BOUTP_outputs/1 -> [BOUTP_outputs]
  BSCP_outputs/1 -> [BSCP_outputs]
  [BSCP_outputs] -> FD5_CE100_0_0x118/1(BSCP_outputs)
  [BOUTP_outputs] -> FD5_CE100_0_0x118/2(BOUTP_outputs)
  FD5_CE100_0_0x118/1(FD5_CE100_0) -> DT_CAN5_SG_FD5_CE100_0/1
  [BSCP_outputs] -> FD5_Debug1_0x4D0/1(BSCP_outputs)
  [BOUTP_outputs] -> FD5_Debug1_0x4D0/2(BOUTP_outputs)
  FD5_Debug1_0x4D0/1(FD5_Debug1) -> DT_CAN5_SG_FD5_Debug1/1
  [BSCP_outputs] -> GW5_CE100_0_0x1C5/1(BSCP_outputs)
  [BOUTP_outputs] -> GW5_CE100_0_0x1C5/2(BOUTP_outputs)
  GW5_CE100_0_0x1C5/1(GW5_CE100_0) -> DT_CAN5_SG_GW5_CE100_0/1

== system halout/HAL_OUT/CAN7 ==
  BOUTP_outputs : Inport  OutDataTypeStr=Bus: BOUTP_outputs
  BSCP_outputs : Inport  Port=2  OutDataTypeStr=Bus: BSCP_outputs
  Trigger : TriggerPort  TriggerType=function-call  VariantControl=(inherit)
  FD7_CE100_0_0x18FA05B9 : Subsystem
  FD7_CE100_1_0xCFFE632 : Subsystem
  DT_CAN7_SG_FD7_CE100_0 : Outport  OutDataTypeStr=Bus: DT_CAN7_SG_FD7_CE100_0
  DT_CAN7_SG_FD7_CE100_1 : Outport  Port=2  OutDataTypeStr=Bus: DT_CAN7_SG_FD7_CE100_1
  wires:
  BOUTP_outputs/1 -> [BOUTP_outputs]
  BSCP_outputs/1 -> [BSCP_outputs]
  [BSCP_outputs] -> FD7_CE100_0_0x18FA05B9/1(BSCP_outputs)
  [BOUTP_outputs] -> FD7_CE100_0_0x18FA05B9/2(BOUTP_outputs)
  FD7_CE100_0_0x18FA05B9/1(FD7_CE100_0) -> DT_CAN7_SG_FD7_CE100_0/1
  [BSCP_outputs] -> FD7_CE100_1_0xCFFE632/1(BSCP_outputs)
  [BOUTP_outputs] -> FD7_CE100_1_0xCFFE632/2(BOUTP_outputs)
  FD7_CE100_1_0xCFFE632/1(FD7_CE100_1) -> DT_CAN7_SG_FD7_CE100_1/1

== system halout/HAL_OUT/CAN1/CCVS_0x18FEF100 ==
  BSCP_outputs : Inport  OutDataTypeStr=Bus: BSCP_outputs
  BOUTP_outputs : Inport  Port=2  OutDataTypeStr=Bus: BOUTP_outputs
  BrakeSW : Subsystem
  ParkBrakeSW : Subsystem
  VCUVehSpd : Subsystem
  bus_creator : BusCreator  Inputs=3  OutDataTypeStr=Bus: DT_CAN1_SG_CCVS  NonVirtualBus=on
  bus_selector : BusSelector  OutputSignals=VOUTP_BrakeSW_enum
  bus_selector1 : BusSelector  OutputSignals=VOUTP_ParkBrakeSW_enum
  bus_selector2 : BusSelector  OutputSignals=VOUTP_VCUVehSpd_kph
  CCVS : Outport
  wires:
  BSCP_outputs/1 -> [BSCP_outputs]
  BOUTP_outputs/1 -> [BOUTP_outputs]
  [CAN1_BrakeSW] -> bus_creator/1  "CAN1_BrakeSW"
  [CAN1_ParkBrakeSW] -> bus_creator/2  "CAN1_ParkBrakeSW"
  [CAN1_VCUVehSpd] -> bus_creator/3  "CAN1_VCUVehSpd"
  bus_creator/1 -> CCVS/1
  BrakeSW/1(CAN1_BrakeSW) -> [CAN1_BrakeSW]
  ParkBrakeSW/1(CAN1_ParkBrakeSW) -> [CAN1_ParkBrakeSW]
  VCUVehSpd/1(CAN1_VCUVehSpd) -> [CAN1_VCUVehSpd]
  bus_selector/1 -> BrakeSW/1(BrakeSW)  "<VOUTP_BrakeSW_enum>"
  [BOUTP_outputs] -> bus_selector/1
  bus_selector1/1 -> ParkBrakeSW/1(ParkBrakeSW)  "<VOUTP_ParkBrakeSW_enum>"
  [BOUTP_outputs] -> bus_selector1/1
  bus_selector2/1 -> VCUVehSpd/1(VCUVehSpd)  "<VOUTP_VCUVehSpd_kph>"
  [BOUTP_outputs] -> bus_selector2/1

== system halout/HAL_OUT/CAN1/CFGEM1_BAM_0x18ECFFEF ==
  BSCP_outputs : Inport  OutDataTypeStr=Bus: BSCP_outputs
  BOUTP_outputs : Inport  Port=2  OutDataTypeStr=Bus: BOUTP_outputs
  CFGEM1BAMPGN : Subsystem
  CFGEM1BAMRsv : Subsystem
  CFGEM1BAMTNum : Subsystem
  CFGEM1BAMTSize : Subsystem
  CFGEM1Ctrl : Subsystem
  bus_creator : BusCreator  Inputs=5  OutDataTypeStr=Bus: DT_CAN1_SG_CFGEM1_BAM  NonVirtualBus=on
  bus_selector : BusSelector  OutputSignals=VOUTP_CFGEM1BAMPGN_raw
  bus_selector1 : BusSelector  OutputSignals=VOUTP_CFGEM1BAMRsv_raw
  bus_selector2 : BusSelector  OutputSignals=VOUTP_CFGEM1BAMTNum_raw
  bus_selector3 : BusSelector  OutputSignals=VOUTP_CFGEM1BAMTSize_raw
  bus_selector4 : BusSelector  OutputSignals=VOUTP_CFGEM1Ctrl_raw
  CFGEM1_BAM : Outport
  wires:
  BSCP_outputs/1 -> [BSCP_outputs]
  BOUTP_outputs/1 -> [BOUTP_outputs]
  [CAN1_CFGEM1BAMPGN] -> bus_creator/1  "CAN1_CFGEM1BAMPGN"
  [CAN1_CFGEM1BAMRsv] -> bus_creator/2  "CAN1_CFGEM1BAMRsv"
  [CAN1_CFGEM1BAMTNum] -> bus_creator/3  "CAN1_CFGEM1BAMTNum"
  [CAN1_CFGEM1BAMTSize] -> bus_creator/4  "CAN1_CFGEM1BAMTSize"
  [CAN1_CFGEM1Ctrl] -> bus_creator/5  "CAN1_CFGEM1Ctrl"
  bus_creator/1 -> CFGEM1_BAM/1
  CFGEM1BAMPGN/1(CAN1_CFGEM1BAMPGN) -> [CAN1_CFGEM1BAMPGN]
  CFGEM1BAMRsv/1(CAN1_CFGEM1BAMRsv) -> [CAN1_CFGEM1BAMRsv]
  CFGEM1BAMTNum/1(CAN1_CFGEM1BAMTNum) -> [CAN1_CFGEM1BAMTNum]
  CFGEM1BAMTSize/1(CAN1_CFGEM1BAMTSize) -> [CAN1_CFGEM1BAMTSize]
  CFGEM1Ctrl/1(CAN1_CFGEM1Ctrl) -> [CAN1_CFGEM1Ctrl]
  bus_selector/1 -> CFGEM1BAMPGN/1(CFGEM1BAMPGN)  "<VOUTP_CFGEM1BAMPGN_raw>"
  [BOUTP_outputs] -> bus_selector/1
  bus_selector1/1 -> CFGEM1BAMRsv/1(CFGEM1BAMRsv)  "<VOUTP_CFGEM1BAMRsv_raw>"
  [BOUTP_outputs] -> bus_selector1/1
  bus_selector2/1 -> CFGEM1BAMTNum/1(CFGEM1BAMTNum)  "<VOUTP_CFGEM1BAMTNum_raw>"
  [BOUTP_outputs] -> bus_selector2/1
  bus_selector3/1 -> CFGEM1BAMTSize/1(CFGEM1BAMTSize)  "<VOUTP_CFGEM1BAMTSize_raw>"
  [BOUTP_outputs] -> bus_selector3/1
  bus_selector4/1 -> CFGEM1Ctrl/1(CFGEM1Ctrl)  "<VOUTP_CFGEM1Ctrl_raw>"
  [BOUTP_outputs] -> bus_selector4/1

== system halout/HAL_OUT/CAN1/CFGEM1_DT_0x18EBFFEF ==
  BSCP_outputs : Inport  OutDataTypeStr=Bus: BSCP_outputs
  BOUTP_outputs : Inport  Port=2  OutDataTypeStr=Bus: BOUTP_outputs
  CFGEM1DT0 : Subsystem
  CFGEM1DT1 : Subsystem
  CFGEM1DT2 : Subsystem
  CFGEM1DT3 : Subsystem
  CFGEM1DT4 : Subsystem
  CFGEM1DT5 : Subsystem
  CFGEM1DT6 : Subsystem
  CFGEM1DT7 : Subsystem
  bus_creator : BusCreator  Inputs=8  OutDataTypeStr=Bus: DT_CAN1_SG_CFGEM1_DT  NonVirtualBus=on
  bus_selector : BusSelector  OutputSignals=VOUTP_DTbyte0_raw
  bus_selector1 : BusSelector  OutputSignals=VOUTP_DTbyte1_raw
  bus_selector2 : BusSelector  OutputSignals=VOUTP_DTbyte2_raw
  bus_selector3 : BusSelector  OutputSignals=VOUTP_DTbyte3_raw
  bus_selector4 : BusSelector  OutputSignals=VOUTP_DTbyte4_raw
  bus_selector5 : BusSelector  OutputSignals=VOUTP_DTbyte5_raw
  bus_selector6 : BusSelector  OutputSignals=VOUTP_DTbyte6_raw
  bus_selector7 : BusSelector  OutputSignals=VOUTP_DTbyte7_raw
  CFGEM1_DT : Outport
  wires:
  BSCP_outputs/1 -> [BSCP_outputs]
  BOUTP_outputs/1 -> [BOUTP_outputs]
  [CAN1_CFGEM1DT0] -> bus_creator/1  "CAN1_CFGEM1DT0"
  [CAN1_CFGEM1DT1] -> bus_creator/2  "CAN1_CFGEM1DT1"
  [CAN1_CFGEM1DT2] -> bus_creator/3  "CAN1_CFGEM1DT2"
  [CAN1_CFGEM1DT3] -> bus_creator/4  "CAN1_CFGEM1DT3"
  [CAN1_CFGEM1DT4] -> bus_creator/5  "CAN1_CFGEM1DT4"
  [CAN1_CFGEM1DT5] -> bus_creator/6  "CAN1_CFGEM1DT5"
  [CAN1_CFGEM1DT6] -> bus_creator/7  "CAN1_CFGEM1DT6"
  [CAN1_CFGEM1DT7] -> bus_creator/8  "CAN1_CFGEM1DT7"
  bus_creator/1 -> CFGEM1_DT/1
  CFGEM1DT0/1(CAN1_CFGEM1DT0) -> [CAN1_CFGEM1DT0]
  CFGEM1DT1/1(CAN1_CFGEM1DT1) -> [CAN1_CFGEM1DT1]
  CFGEM1DT2/1(CAN1_CFGEM1DT2) -> [CAN1_CFGEM1DT2]
  CFGEM1DT3/1(CAN1_CFGEM1DT3) -> [CAN1_CFGEM1DT3]
  CFGEM1DT4/1(CAN1_CFGEM1DT4) -> [CAN1_CFGEM1DT4]
  CFGEM1DT5/1(CAN1_CFGEM1DT5) -> [CAN1_CFGEM1DT5]
  CFGEM1DT6/1(CAN1_CFGEM1DT6) -> [CAN1_CFGEM1DT6]
  CFGEM1DT7/1(CAN1_CFGEM1DT7) -> [CAN1_CFGEM1DT7]
  bus_selector/1 -> CFGEM1DT0/1(CFGEM1DT0)  "<VOUTP_DTbyte0_raw>"
  [BOUTP_outputs] -> bus_selector/1
  bus_selector1/1 -> CFGEM1DT1/1(CFGEM1DT1)  "<VOUTP_DTbyte1_raw>"
  [BOUTP_outputs] -> bus_selector1/1
  bus_selector2/1 -> CFGEM1DT2/1(CFGEM1DT2)  "<VOUTP_DTbyte2_raw>"
  [BOUTP_outputs] -> bus_selector2/1
  bus_selector3/1 -> CFGEM1DT3/1(CFGEM1DT3)  "<VOUTP_DTbyte3_raw>"
  [BOUTP_outputs] -> bus_selector3/1
  bus_selector4/1 -> CFGEM1DT4/1(CFGEM1DT4)  "<VOUTP_DTbyte4_raw>"
  [BOUTP_outputs] -> bus_selector4/1
  bus_selector5/1 -> CFGEM1DT5/1(CFGEM1DT5)  "<VOUTP_DTbyte5_raw>"
  [BOUTP_outputs] -> bus_selector5/1
  bus_selector6/1 -> CFGEM1DT6/1(CFGEM1DT6)  "<VOUTP_DTbyte6_raw>"
  [BOUTP_outputs] -> bus_selector6/1
  bus_selector7/1 -> CFGEM1DT7/1(CFGEM1DT7)  "<VOUTP_DTbyte7_raw>"
  [BOUTP_outputs] -> bus_selector7/1

== system halout/HAL_OUT/CAN1/EEC2_0xCF00300 ==
  BSCP_outputs : Inport  OutDataTypeStr=Bus: BSCP_outputs
  BOUTP_outputs : Inport  Port=2  OutDataTypeStr=Bus: BOUTP_outputs
  AccPedal1LowSW : Subsystem
  AccPedalPos1 : Subsystem
  EEC2MSGCS : Subsystem
  EEC2MSGCnt : Subsystem
  bus_creator : BusCreator  Inputs=4  OutDataTypeStr=Bus: DT_CAN1_SG_EEC2  NonVirtualBus=on
  bus_selector : BusSelector  OutputSignals=VOUTP_AccPedal1LowSW_enum
  bus_selector1 : BusSelector  OutputSignals=VOUTP_AccPedalPos1_pct
  bus_selector2 : BusSelector  OutputSignals=VOUTP_EEC2MSGCS_raw
  bus_selector3 : BusSelector  OutputSignals=VOUTP_EEC2MSGCnt_raw
  EEC2 : Outport
  wires:
  BSCP_outputs/1 -> [BSCP_outputs]
  BOUTP_outputs/1 -> [BOUTP_outputs]
  [CAN1_AccPedal1LowSW] -> bus_creator/1  "CAN1_AccPedal1LowSW"
  [CAN1_AccPedalPos1] -> bus_creator/2  "CAN1_AccPedalPos1"
  [CAN1_EEC2MSGCS] -> bus_creator/3  "CAN1_EEC2MSGCS"
  [CAN1_EEC2MSGCnt] -> bus_creator/4  "CAN1_EEC2MSGCnt"
  bus_creator/1 -> EEC2/1
  AccPedal1LowSW/1(CAN1_AccPedal1LowSW) -> [CAN1_AccPedal1LowSW]
  AccPedalPos1/1(CAN1_AccPedalPos1) -> [CAN1_AccPedalPos1]
  EEC2MSGCS/1(CAN1_EEC2MSGCS) -> [CAN1_EEC2MSGCS]
  EEC2MSGCnt/1(CAN1_EEC2MSGCnt) -> [CAN1_EEC2MSGCnt]
  bus_selector/1 -> AccPedal1LowSW/1(AccPedal1LowSW)  "<VOUTP_AccPedal1LowSW_enum>"
  [BOUTP_outputs] -> bus_selector/1
  bus_selector1/1 -> AccPedalPos1/1(AccPedalPos1)  "<VOUTP_AccPedalPos1_pct>"
  [BOUTP_outputs] -> bus_selector1/1
  bus_selector2/1 -> EEC2MSGCS/1(EEC2MSGCS)  "<VOUTP_EEC2MSGCS_raw>"
  [BOUTP_outputs] -> bus_selector2/1
  bus_selector3/1 -> EEC2MSGCnt/1(EEC2MSGCnt)  "<VOUTP_EEC2MSGCnt_raw>"
  [BOUTP_outputs] -> bus_selector3/1

== system halout/HAL_OUT/CAN1/EEC3_0x18FEDFEF ==
  BSCP_outputs : Inport  OutDataTypeStr=Bus: BSCP_outputs
  BOUTP_outputs : Inport  Port=2  OutDataTypeStr=Bus: BOUTP_outputs
  EMParasLoss : Subsystem
  NFricPercTorq : Subsystem
  bus_creator : BusCreator  Inputs=2  OutDataTypeStr=Bus: DT_CAN1_SG_EEC3  NonVirtualBus=on
  bus_selector : BusSelector  OutputSignals=VOUTP_EMParasLoss_pct
  bus_selector1 : BusSelector  OutputSignals=VOUTP_NFricPercTorq_pct
  EEC3 : Outport
  wires:
  BSCP_outputs/1 -> [BSCP_outputs]
  BOUTP_outputs/1 -> [BOUTP_outputs]
  [CAN1_EMParasLoss] -> bus_creator/1  "CAN1_EMParasLoss"
  [CAN1_NFricPercTorq] -> bus_creator/2  "CAN1_NFricPercTorq"
  bus_creator/1 -> EEC3/1
  EMParasLoss/1(CAN1_EMParasLoss) -> [CAN1_EMParasLoss]
  NFricPercTorq/1(CAN1_NFricPercTorq) -> [CAN1_NFricPercTorq]
  bus_selector/1 -> EMParasLoss/1(EMParasLoss)  "<VOUTP_EMParasLoss_pct>"
  [BOUTP_outputs] -> bus_selector/1
  bus_selector1/1 -> NFricPercTorq/1(NFricPercTorq)  "<VOUTP_NFricPercTorq_pct>"
  [BOUTP_outputs] -> bus_selector1/1

== system halout/HAL_OUT/CAN1/EMRC1_0x18FF20EF ==
  BSCP_outputs : Inport  OutDataTypeStr=Bus: BSCP_outputs
  BOUTP_outputs : Inport  Port=2  OutDataTypeStr=Bus: BOUTP_outputs
  ActEMOutSftSpd : Subsystem
  ActEMpTrq : Subsystem
  ActEMpTrqHrls : Subsystem
  ActMaxAvaEMRecpTrq : Subsystem
  DrvDemEMRtapTrq : Subsystem
  EMTrqModeDrvBrk : Subsystem
  RetSelNonEng : Subsystem
  SACtrlDev : Subsystem
  bus_creator : BusCreator  Inputs=8  OutDataTypeStr=Bus: DT_CAN1_SG_EMRC1  NonVirtualBus=on
  bus_selector : BusSelector  OutputSignals=VOUTP_ActEMOutSftSpd_rpm
  bus_selector1 : BusSelector  OutputSignals=VOUTP_ActEMpTrq_pct
  bus_selector2 : BusSelector  OutputSignals=VOUTP_ActEMpTrqHrls_pct
  bus_selector3 : BusSelector  OutputSignals=VOUTP_ActMaxAvaEMRecpTrq_pct
  bus_selector4 : BusSelector  OutputSignals=VOUTP_DrvDemEMRtapTrq_pct
  bus_selector5 : BusSelector  OutputSignals=VOUTP_EMTrqModeDrvBrk_enum
  bus_selector6 : BusSelector  OutputSignals=VOUTP_RetSelNonEng_pct
  bus_selector7 : BusSelector  OutputSignals=VOUTP_SACtrlDev_enum
  EMRC1 : Outport
  wires:
  BSCP_outputs/1 -> [BSCP_outputs]
  BOUTP_outputs/1 -> [BOUTP_outputs]
  [CAN1_ActEMOutSftSpd] -> bus_creator/1  "CAN1_ActEMOutSftSpd"
  [CAN1_ActEMpTrq] -> bus_creator/2  "CAN1_ActEMpTrq"
  [CAN1_ActEMpTrqHrls] -> bus_creator/3  "CAN1_ActEMpTrqHrls"
  [CAN1_ActMaxAvaEMRecpTrq] -> bus_creator/4  "CAN1_ActMaxAvaEMRecpTrq"
  [CAN1_DrvDemEMRtapTrq] -> bus_creator/5  "CAN1_DrvDemEMRtapTrq"
  [CAN1_EMTrqModeDrvBrk] -> bus_creator/6  "CAN1_EMTrqModeDrvBrk"
  [CAN1_RetSelNonEng] -> bus_creator/7  "CAN1_RetSelNonEng"
  [CAN1_SACtrlDev] -> bus_creator/8  "CAN1_SACtrlDev"
  bus_creator/1 -> EMRC1/1
  ActEMOutSftSpd/1(CAN1_ActEMOutSftSpd) -> [CAN1_ActEMOutSftSpd]
  ActEMpTrq/1(CAN1_ActEMpTrq) -> [CAN1_ActEMpTrq]
  ActEMpTrqHrls/1(CAN1_ActEMpTrqHrls) -> [CAN1_ActEMpTrqHrls]
  ActMaxAvaEMRecpTrq/1(CAN1_ActMaxAvaEMRecpTrq) -> [CAN1_ActMaxAvaEMRecpTrq]
  DrvDemEMRtapTrq/1(CAN1_DrvDemEMRtapTrq) -> [CAN1_DrvDemEMRtapTrq]
  EMTrqModeDrvBrk/1(CAN1_EMTrqModeDrvBrk) -> [CAN1_EMTrqModeDrvBrk]
  RetSelNonEng/1(CAN1_RetSelNonEng) -> [CAN1_RetSelNonEng]
  SACtrlDev/1(CAN1_SACtrlDev) -> [CAN1_SACtrlDev]
  bus_selector/1 -> ActEMOutSftSpd/1(ActEMOutSftSpd)  "<VOUTP_ActEMOutSftSpd_rpm>"
  [BOUTP_outputs] -> bus_selector/1
  bus_selector1/1 -> ActEMpTrq/1(ActEMpTrq)  "<VOUTP_ActEMpTrq_pct>"
  [BOUTP_outputs] -> bus_selector1/1
  bus_selector2/1 -> ActEMpTrqHrls/1(ActEMpTrqHrls)  "<VOUTP_ActEMpTrqHrls_pct>"
  [BOUTP_outputs] -> bus_selector2/1
  bus_selector3/1 -> ActMaxAvaEMRecpTrq/1(ActMaxAvaEMRecpTrq)  "<VOUTP_ActMaxAvaEMRecpTrq_pct>"
  [BOUTP_outputs] -> bus_selector3/1
  bus_selector4/1 -> DrvDemEMRtapTrq/1(DrvDemEMRtapTrq)  "<VOUTP_DrvDemEMRtapTrq_pct>"
  [BOUTP_outputs] -> bus_selector4/1
  bus_selector5/1 -> EMTrqModeDrvBrk/1(EMTrqModeDrvBrk)  "<VOUTP_EMTrqModeDrvBrk_enum>"
  [BOUTP_outputs] -> bus_selector5/1
  bus_selector6/1 -> RetSelNonEng/1(RetSelNonEng)  "<VOUTP_RetSelNonEng_pct>"
  [BOUTP_outputs] -> bus_selector6/1
  bus_selector7/1 -> SACtrlDev/1(SACtrlDev)  "<VOUTP_SACtrlDev_enum>"
  [BOUTP_outputs] -> bus_selector7/1

== system halout/HAL_OUT/CAN1/ETC1_0x18F00203 ==
  BSCP_outputs : Inport  OutDataTypeStr=Bus: BSCP_outputs
  BOUTP_outputs : Inport  Port=2  OutDataTypeStr=Bus: BOUTP_outputs
  DLEngaged : Subsystem
  ShiftPgs : Subsystem
  bus_creator : BusCreator  Inputs=2  OutDataTypeStr=Bus: DT_CAN1_SG_ETC1  NonVirtualBus=on
  bus_selector : BusSelector  OutputSignals=VOUTP_DLEngaged_enum
  bus_selector1 : BusSelector  OutputSignals=VOUTP_ShiftPgs_enum
  ETC1 : Outport
  wires:
  BSCP_outputs/1 -> [BSCP_outputs]
  BOUTP_outputs/1 -> [BOUTP_outputs]
  [CAN1_DLEngaged] -> bus_creator/1  "CAN1_DLEngaged"
  [CAN1_ShiftPgs] -> bus_creator/2  "CAN1_ShiftPgs"
  bus_creator/1 -> ETC1/1
  DLEngaged/1(CAN1_DLEngaged) -> [CAN1_DLEngaged]
  ShiftPgs/1(CAN1_ShiftPgs) -> [CAN1_ShiftPgs]
  bus_selector/1 -> DLEngaged/1(DLEngaged)  "<VOUTP_DLEngaged_enum>"
  [BOUTP_outputs] -> bus_selector/1
  bus_selector1/1 -> ShiftPgs/1(ShiftPgs)  "<VOUTP_ShiftPgs_enum>"
  [BOUTP_outputs] -> bus_selector1/1

== system halout/HAL_OUT/CAN1/ETC2_0x18F00503 ==
  BSCP_outputs : Inport  OutDataTypeStr=Bus: BSCP_outputs
  BOUTP_outputs : Inport  Port=2  OutDataTypeStr=Bus: BOUTP_outputs
  ActDriveDirect : Subsystem
  bus_creator : BusCreator  Inputs=1  OutDataTypeStr=Bus: DT_CAN1_SG_ETC2  NonVirtualBus=on
  bus_selector : BusSelector  OutputSignals=VOUTP_ActDriveDirect_enum
  ETC2 : Outport
  wires:
  BSCP_outputs/1 -> [BSCP_outputs]
  BOUTP_outputs/1 -> [BOUTP_outputs]
  [CAN1_ActDriveDirect] -> bus_creator/1  "CAN1_ActDriveDirect"
  bus_creator/1 -> ETC2/1
  ActDriveDirect/1(CAN1_ActDriveDirect) -> [CAN1_ActDriveDirect]
  bus_selector/1 -> ActDriveDirect/1(ActDriveDirect)  "<VOUTP_ActDriveDirect_enum>"
  [BOUTP_outputs] -> bus_selector/1

== system halout/HAL_OUT/CAN1/FD1_C100_1_0x18FF602B ==
  BSCP_outputs : Inport  OutDataTypeStr=Bus: BSCP_outputs
  BOUTP_outputs : Inport  Port=2  OutDataTypeStr=Bus: BOUTP_outputs
  FDCCHAEBSHBSwSta : Subsystem
  FDCCHAEBSHHSwSta : Subsystem
  bus_creator : BusCreator  Inputs=2  OutDataTypeStr=Bus: DT_CAN1_SG_FD1_C100_1  NonVirtualBus=on
  bus_selector : BusSelector  OutputSignals=VOUTP_FDCCHAEBSHBSwSta_enum
  bus_selector1 : BusSelector  OutputSignals=VOUTP_FDCCHAEBSHHSwSta_enum
  FD1_C100_1 : Outport
  wires:
  BSCP_outputs/1 -> [BSCP_outputs]
  BOUTP_outputs/1 -> [BOUTP_outputs]
  [CAN1_FDC_CHA_EBSHBSw_Sta] -> bus_creator/1  "CAN1_FDC_CHA_EBSHBSw_Sta"
  [CAN1_FDC_CHA_EBSHHSw_Sta] -> bus_creator/2  "CAN1_FDC_CHA_EBSHHSw_Sta"
  bus_creator/1 -> FD1_C100_1/1
  FDCCHAEBSHBSwSta/1(CAN1_FDC_CHA_EBSHBSw_Sta) -> [CAN1_FDC_CHA_EBSHBSw_Sta]
  FDCCHAEBSHHSwSta/1(CAN1_FDC_CHA_EBSHHSw_Sta) -> [CAN1_FDC_CHA_EBSHHSw_Sta]
  bus_selector/1 -> FDCCHAEBSHBSwSta/1(FDCCHAEBSHBSwSta)  "<VOUTP_FDCCHAEBSHBSwSta_enum>"
  [BOUTP_outputs] -> bus_selector/1
  bus_selector1/1 -> FDCCHAEBSHHSwSta/1(FDCCHAEBSHHSwSta)  "<VOUTP_FDCCHAEBSHHSwSta_enum>"
  [BOUTP_outputs] -> bus_selector1/1

== system halout/HAL_OUT/CAN1/FD1_C100_2_0x18FE4A03 ==
  BSCP_outputs : Inport  OutDataTypeStr=Bus: BSCP_outputs
  BOUTP_outputs : Inport  Port=2  OutDataTypeStr=Bus: BOUTP_outputs
  FDCCHAEBSRd4BRSta : Subsystem
  bus_creator : BusCreator  Inputs=1  OutDataTypeStr=Bus: DT_CAN1_SG_FD1_C100_2  NonVirtualBus=on
  bus_selector : BusSelector  OutputSignals=VOUTP_FDCCHAEBSRd4BRSta_enum
  FD1_C100_2 : Outport
  wires:
  BSCP_outputs/1 -> [BSCP_outputs]
  BOUTP_outputs/1 -> [BOUTP_outputs]
  [CAN1_FDC_CHA_EBSRd4BR_Sta] -> bus_creator/1  "CAN1_FDC_CHA_EBSRd4BR_Sta"
  bus_creator/1 -> FD1_C100_2/1
  FDCCHAEBSRd4BRSta/1(CAN1_FDC_CHA_EBSRd4BR_Sta) -> [CAN1_FDC_CHA_EBSRd4BR_Sta]
  bus_selector/1 -> FDCCHAEBSRd4BRSta/1(FDCCHAEBSRd4BRSta)  "<VOUTP_FDCCHAEBSRd4BRSta_enum>"
  [BOUTP_outputs] -> bus_selector/1

== system halout/HAL_OUT/CAN1/FD1_C100_3_0xCF103D0 ==
  BSCP_outputs : Inport  OutDataTypeStr=Bus: BSCP_outputs
  BOUTP_outputs : Inport  Port=2  OutDataTypeStr=Bus: BOUTP_outputs
  DCDCEnDemand : Subsystem
  EACSpdDemand : Subsystem
  EHPSEnDemand : Subsystem
  EHPSSpdDemand : Subsystem
  FDCCHAEACEnDemandCmd : Subsystem
  Ground : Ground
  Ground1 : Ground
  bus_creator : BusCreator  Inputs=5  OutDataTypeStr=Bus: DT_CAN1_SG_FD1_C100_3  NonVirtualBus=on
  bus_selector : BusSelector  OutputSignals=VOUTP_DCDCEnDem_enum
  bus_selector1 : BusSelector  OutputSignals=VOUTP_EHPSEnDem_enum
  bus_selector2 : BusSelector  OutputSignals=VOUTP_EACEnDem_enum
  FD1_C100_3 : Outport
  wires:
  BSCP_outputs/1 -> [BSCP_outputs]
  BOUTP_outputs/1 -> [BOUTP_outputs]
  [CAN1_DCDCEnDemand] -> bus_creator/1  "CAN1_DCDCEnDemand"
  [CAN1_EACSpdDemand] -> bus_creator/2  "CAN1_EACSpdDemand"
  [CAN1_EHPSEnDemand] -> bus_creator/3  "CAN1_EHPSEnDemand"
  [CAN1_EHPSSpdDemand] -> bus_creator/4  "CAN1_EHPSSpdDemand"
  [CAN1_FDC_CHA_EACEnDemand_Cmd] -> bus_creator/5  "CAN1_FDC_CHA_EACEnDemand_Cmd"
  bus_creator/1 -> FD1_C100_3/1
  DCDCEnDemand/1(CAN1_DCDCEnDemand) -> [CAN1_DCDCEnDemand]
  EACSpdDemand/1(CAN1_EACSpdDemand) -> [CAN1_EACSpdDemand]
  EHPSEnDemand/1(CAN1_EHPSEnDemand) -> [CAN1_EHPSEnDemand]
  EHPSSpdDemand/1(CAN1_EHPSSpdDemand) -> [CAN1_EHPSSpdDemand]
  FDCCHAEACEnDemandCmd/1(CAN1_FDC_CHA_EACEnDemand_Cmd) -> [CAN1_FDC_CHA_EACEnDemand_Cmd]
  bus_selector/1 -> DCDCEnDemand/1(DCDCEnDemand)  "<VOUTP_DCDCEnDem_enum>"
  [BOUTP_outputs] -> bus_selector/1
  Ground/1 -> EACSpdDemand/1(EACSpdDemand)
  bus_selector1/1 -> EHPSEnDemand/1(EHPSEnDemand)  "<VOUTP_EHPSEnDem_enum>"
  [BOUTP_outputs] -> bus_selector1/1
  Ground1/1 -> EHPSSpdDemand/1(EHPSSpdDemand)
  bus_selector2/1 -> FDCCHAEACEnDemandCmd/1(FDCCHAEACEnDemandCmd)  "<VOUTP_EACEnDem_enum>"
  [BOUTP_outputs] -> bus_selector2/1

== system halout/HAL_OUT/CAN1/FD1_CE100_1_0x18FE4EEC ==
  BSCP_outputs : Inport  OutDataTypeStr=Bus: BSCP_outputs
  BOUTP_outputs : Inport  Port=2  OutDataTypeStr=Bus: BOUTP_outputs
  FDCBCMDoorStaSta : Subsystem
  bus_creator : BusCreator  Inputs=1  OutDataTypeStr=Bus: DT_CAN1_SG_FD1_CE100_1  NonVirtualBus=on
  bus_selector : BusSelector  OutputSignals=VOUTP_DoorStaSta_enum
  FD1_CE100_1 : Outport
  wires:
  BSCP_outputs/1 -> [BSCP_outputs]
  BOUTP_outputs/1 -> [BOUTP_outputs]
  [CAN1_FDC_BCM_DoorSta_Sta] -> bus_creator/1  "CAN1_FDC_BCM_DoorSta_Sta"
  bus_creator/1 -> FD1_CE100_1/1
  FDCBCMDoorStaSta/1(CAN1_FDC_BCM_DoorSta_Sta) -> [CAN1_FDC_BCM_DoorSta_Sta]
  bus_selector/1 -> FDCBCMDoorStaSta/1(FDCBCMDoorStaSta)  "<VOUTP_DoorStaSta_enum>"
  [BOUTP_outputs] -> bus_selector/1
